simulink model "VVI"  (R2022b)
settings: Solver=FixedStepAuto  StartTime=0.0  StopTime=10.0  FixedStep=1e-3  RelTol=1e-3  EnableMultiTasking=on
undefined symbols (not defined in the file): D0, D1, D10, D11, D12, D13, D2, D3, D5, D8, D9, PTA0, PTA1, PTA2, PTB9, PTC16, PTC17, PTC4, PTD0, PTD1, PTD2, PTD3
libraries: frdmk64flib x14
settings Model: ExtModeTrigDuration=5  Creator=jathe  LastModifiedBy=mutha
settings SolverCC: AlgebraicLoopSolver=TrustRegion
settings OptimizationCC: EnhancedBackFolding=on  PassReuseOutputArgsAs=Individual arguments  ZeroExternalMemoryAtStartup=off  ZeroInternalMemoryAtStartup=off  MaxStackSize=64  OptimizeBlockOrder=speed  DifferentSizesBufferReuse=on  OptimizationCustomize=off  EfficientTunableParamExpr=on
settings DebuggingCC: ParameterTunabilityLossMsg=error  UnconnectedInputMsg=warning  UnconnectedOutputMsg=warning  UnconnectedLineMsg=warning  SFMachineParentedDataDiag=warning
settings HardwareCC: ProdBitPerPointer=32  ProdBitPerSizeT=32  ProdBitPerPtrDiffT=32  ProdLargestAtomicInteger=Long  ProdLargestAtomicFloat=Double  ProdWordSize=32  ProdHWDeviceType=ARM Compatible->ARM Cortex
settings ModelReferenceCC: EnableRefExpFcnMdlSchedulingChecks=on
settings SFSimCC: MATLABDynamicMemAlloc=off
settings RTWCC: Description=Embedded Coder  SystemTargetFile=ert.tlc  HardwareBoard=NXP FRDM-K64F  TLCOptions="-aInlineSetEventsForThisBaseRateFcn=TLC_FALSE -aSuppressMultiTaskScheduler=TLC_FALSE  -aRateBasedStepFcn=0"  TemplateMakefile=ert_default_tmf  Toolchain=GNU Tools for ARM Embedded Processors  DLArmComputeVersion=19.05
settings CodeAppCC: ForceParamTrailComments=on  IgnoreCustomStorageClasses=off  OperatorAnnotations=on  SimulinkDataObjDesc=on  SFDataObjDesc=on  InsertBlockDesc=on
settings ERTTargetCC: ExtModeTransport=4  ExtModeMexFile=sendToCommService

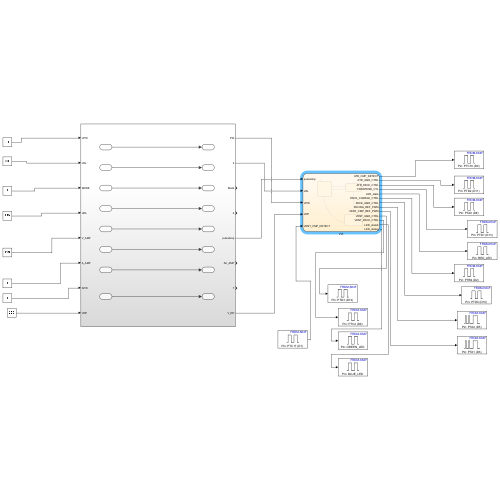
[thumbnail: Simulink's stored preview of the top-level diagram]
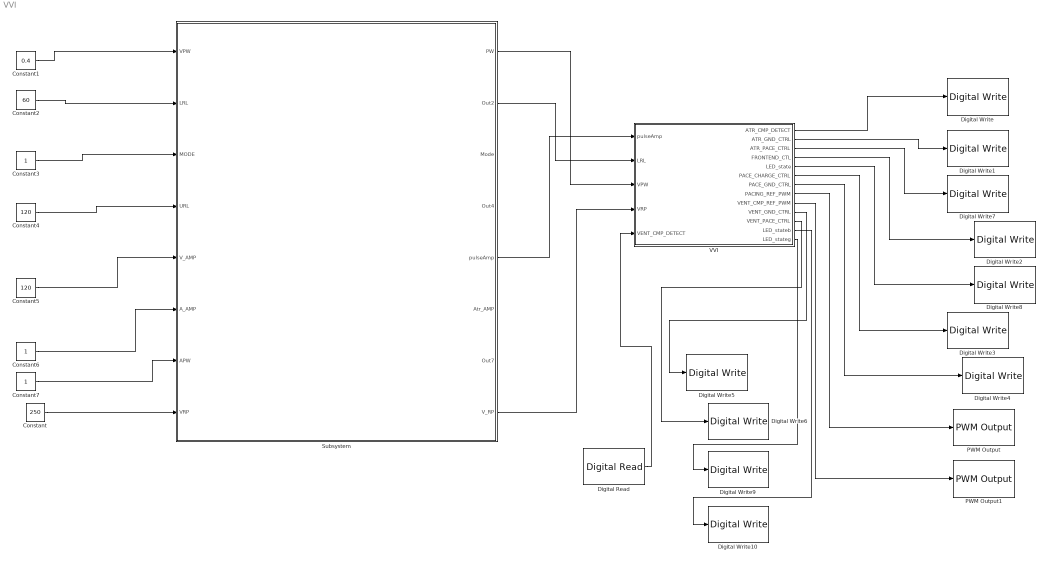
== system VVI ==
  Constant : Constant  Value=250  OutDataTypeStr=int16
  Constant1 : Constant  Value=0.4  OutDataTypeStr=int16
  Constant2 : Constant  Value=60  OutDataTypeStr=int16
  Constant3 : Constant  OutDataTypeStr=int16
  Constant4 : Constant  Value=120  OutDataTypeStr=int16
  Constant5 : Constant  Value=120  OutDataTypeStr=int16
  Constant6 : Constant  OutDataTypeStr=int16
  Constant7 : Constant  OutDataTypeStr=int16
  Digital Read : frdmk64flib/Digital Read  Whichpin=PTC17 (D1)  SampleTime=-1
  Digital Write : frdmk64flib/Digital Write  Whichpin=PTC16 (D0)
  Digital Write1 : frdmk64flib/Digital Write  Whichpin=PTD2 (D11)
  Digital Write10 : frdmk64flib/Digital Write  Whichpin=BLUE_LED
  Digital Write2 : frdmk64flib/Digital Write  Whichpin=PTD1 (D13)
  Digital Write3 : frdmk64flib/Digital Write  Whichpin=PTB9 (D2)
  Digital Write4 : frdmk64flib/Digital Write  Whichpin=PTD0 (D10)
  Digital Write5 : frdmk64flib/Digital Write  Whichpin=PTD3 (D12)
  Digital Write6 : frdmk64flib/Digital Write  Whichpin=PTC4 (D9)
  Digital Write7 : frdmk64flib/Digital Write  Whichpin=PTA0 (D8)
  Digital Write8 : frdmk64flib/Digital Write  Whichpin=RED_LED
  Digital Write9 : frdmk64flib/Digital Write  Whichpin=GREEN_LED
  PWM Output : frdmk64flib/PWM Output  Whichpin=PTA2 (D5)  InitialFrequency=2000  InitialDutyCycle=0
  PWM Output1 : frdmk64flib/PWM Output  Whichpin=PTA1 (D3)  InitialFrequency=2000  InitialDutyCycle=0
  Subsystem : Subsystem
  VVI : Stateflow chart  TreatAsAtomicUnit=on
  wires:
  Constant4/1 -> Subsystem/4(URL)
  Constant6/1 -> Subsystem/6(A_AMP)
  Constant5/1 -> Subsystem/5(V_AMP)
  Constant2/1 -> Subsystem/2(LRL)
  Constant3/1 -> Subsystem/3(MODE)
  Constant1/1 -> Subsystem/1(VPW)
  Constant7/1 -> Subsystem/7(APW)
  Subsystem/5(pulseAmp) -> VVI/1(pulseAmp)
  Subsystem/2(Out2) -> VVI/2(LRL)
  Subsystem/1(PW) -> VVI/3(VPW)
  Constant/1 -> Subsystem/8(VRP)
  Subsystem/8(V_RP) -> VVI/4(VRP)
  VVI/1(ATR_CMP_DETECT) -> Digital Write/1
  VVI/2(ATR_GND_CTRL) -> Digital Write1/1
  VVI/3(ATR_PACE_CTRL) -> Digital Write7/1
  VVI/4(FRONTEND_CTL) -> Digital Write2/1
  VVI/5(LED_state) -> Digital Write8/1
  VVI/6(PACE_CHARGE_CTRL) -> Digital Write3/1
  VVI/7(PACE_GND_CTRL) -> Digital Write4/1
  VVI/8(PACING_REF_PWM) -> PWM Output/1
  VVI/9(VENT_CMP_REF_PWM) -> PWM Output1/1
  VVI/10(VENT_GND_CTRL) -> Digital Write5/1
  VVI/11(VENT_PACE_CTRL) -> Digital Write6/1
  Digital Read/1 -> VVI/5(VENT_CMP_DETECT)
  VVI/13(LED_stateg) -> Digital Write9/1
  VVI/12(LED_stateb) -> Digital Write10/1

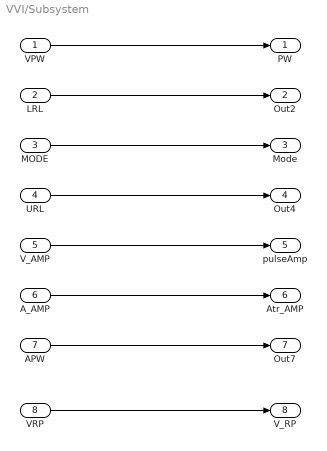
== system VVI/Subsystem ==
  VPW : Inport  OutDataTypeStr=int16
  LRL : Inport  Port=2  OutDataTypeStr=int16
  MODE : Inport  Port=3
  URL : Inport  Port=4  OutDataTypeStr=int16
  V_AMP : Inport  Port=5  OutDataTypeStr=int16
  A_AMP : Inport  Port=6  OutDataTypeStr=int16
  APW : Inport  Port=7  OutDataTypeStr=int16
  VRP : Inport  Port=8  OutDataTypeStr=int16
  PW : Outport
  Out2 : Outport  Port=2
  Mode : Outport  Port=3
  Out4 : Outport  Port=4
  pulseAmp : Outport  Port=5
  Atr_AMP : Outport  Port=6
  Out7 : Outport  Port=7
  V_RP : Outport  Port=8
  wires:
  VPW/1 -> PW/1
  LRL/1 -> Out2/1
  MODE/1 -> Mode/1
  URL/1 -> Out4/1
  V_AMP/1 -> pulseAmp/1
  A_AMP/1 -> Atr_AMP/1
  APW/1 -> Out7/1
  VRP/1 -> V_RP/1

== stateflow chart VVI/VVI ==
  state SETUP_VENT_SENSE %State 1(VOO)
    entry:
    FRONTEND_CTL = true;
    PACING_REF_PWM = 40;
    %(pulseAmp/5)
    VENT_CMP_REF_PWM = 53;
    PACE_GND_CTRL = true;
    ATR_CMP_DETECT = false;
    PACE_CHARGE_CTRL = true;
    VENT_PACE_CTRL = false;
    VENT_GND_CTRL = true;
    ATR_PACE_CTRL = false;
    ATR_GND_CTRL = false;
    LED_state=false;
    LED_stateb=false;
    LED_stateg=false;
  state SENSE_PULSE %Start sensing after VRP
    entry:
    LED_state=false;
    LED_stateb=true;
    LED_stateg=false;
  state VENT_PACE_PT2 %Discharging C22
    entry:
    PACE_CHARGE_CTRL = false;
    VENT_PACE_CTRL = true;
    VENT_GND_CTRL = false; %not sure
    %LED STATE
    LED_state=true;
    LED_stateb=false;
    LED_stateg=false;
  (default) -> SETUP_VENT_SENSE %State 1(VOO)
  SETUP_VENT_SENSE %State 1(VOO) -> SENSE_PULSE %Start sensing after VRP : after(VRP, msec)
  SENSE_PULSE %Start sensing after VRP -> SETUP_VENT_SENSE %State 1(VOO) [order 2] : [(VENT_CMP_DETECT == true)]
  SENSE_PULSE %Start sensing after VRP -> VENT_PACE_PT2 %Discharging C22 [order 1] : after((60000/LRL) - VRP, msec)
  VENT_PACE_PT2 %Discharging C22 -> SETUP_VENT_SENSE %State 1(VOO) : after(VPW,msec)
  data: pulseAmp input int16; ATR_CMP_DETECT output boolean; ATR_GND_CTRL output boolean; ATR_PACE_CTRL output boolean; FRONTEND_CTL output boolean; LED_state output boolean; PACE_CHARGE_CTRL output boolean; PACE_GND_CTRL output boolean; PACING_REF_PWM output int16; VENT_CMP_REF_PWM output int16; VENT_GND_CTRL output boolean; VENT_PACE_CTRL output boolean; LRL input int16; VPW input int16; VRP input int16; VENT_CMP_DETECT input boolean; LED_stateb output; LED_stateg output
